simulink model "Group44VVI"  (R2022b)
settings: Solver=FixedStepAuto  StartTime=0.0  StopTime=10.0  FixedStep=1e-3  RelTol=1e-3  EnableMultiTasking=on
undefined symbols (not defined in the file): D1, D10, D11, D12, D2, D3, D4, D5, D7, D8, D9, PTA0, PTA1, PTA2, PTB23, PTB9, PTC17, PTC3, PTC4, PTD0, PTD2, PTD3
libraries: frdmk64flib x11
settings Model: ExtModeTrigDuration=5  Creator=Admin  LastModifiedBy=Admin
settings OptimizationCC: EnhancedBackFolding=on  PassReuseOutputArgsAs=Individual arguments  ZeroExternalMemoryAtStartup=off  ZeroInternalMemoryAtStartup=off  MaxStackSize=64  OptimizeBlockOrder=speed  DifferentSizesBufferReuse=on  OptimizationCustomize=off  EfficientTunableParamExpr=on
settings DebuggingCC: ParameterTunabilityLossMsg=error
settings HardwareCC: ProdBitPerPointer=32  ProdBitPerSizeT=32  ProdBitPerPtrDiffT=32  ProdLargestAtomicInteger=Long  ProdLargestAtomicFloat=Double  ProdWordSize=32  ProdHWDeviceType=ARM Compatible->ARM Cortex
settings SFSimCC: MATLABDynamicMemAlloc=off
settings RTWCC: Description=Embedded Coder  SystemTargetFile=ert.tlc  HardwareBoard=NXP FRDM-K64F  TLCOptions="-aInlineSetEventsForThisBaseRateFcn=TLC_FALSE -aSuppressMultiTaskScheduler=TLC_FALSE  -aRateBasedStepFcn=0"  TemplateMakefile=ert_default_tmf  Toolchain=GNU Tools for ARM Embedded Processors
settings CodeAppCC: ForceParamTrailComments=on  IgnoreCustomStorageClasses=off  OperatorAnnotations=on  SimulinkDataObjDesc=on  SFDataObjDesc=on  InsertBlockDesc=on
settings ERTTargetCC: ExtModeTransport=4  ExtModeMexFile=sendToCommService

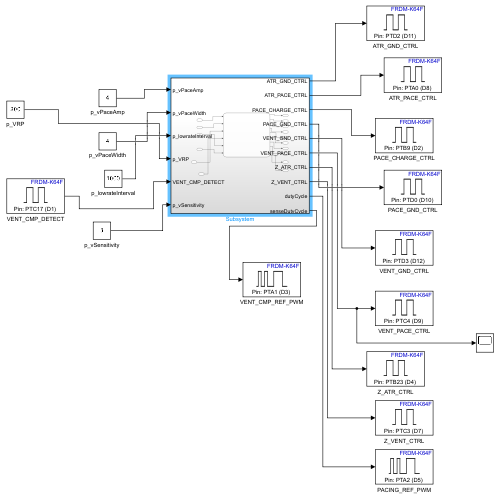
[thumbnail: Simulink's stored preview of the top-level diagram]
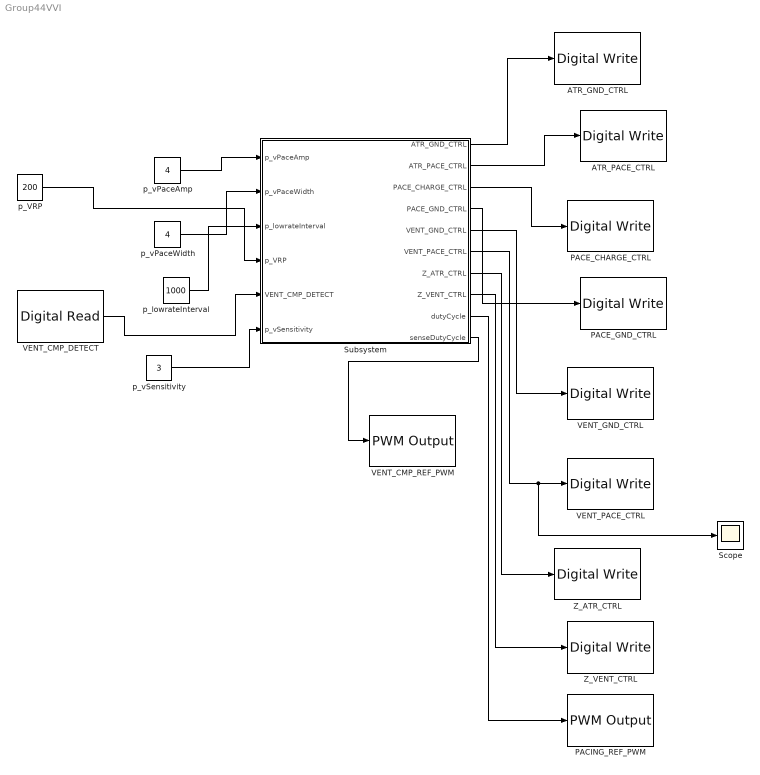
== system Group44VVI ==
  ATR_GND_CTRL : frdmk64flib/Digital Write  Whichpin=PTD2 (D11)
  ATR_PACE_CTRL : frdmk64flib/Digital Write  Whichpin=PTA0 (D8)
  PACE_CHARGE_CTRL : frdmk64flib/Digital Write  Whichpin=PTB9 (D2)
  PACE_GND_CTRL : frdmk64flib/Digital Write  Whichpin=PTD0 (D10)
  PACING_REF_PWM : frdmk64flib/PWM Output  Whichpin=PTA2 (D5)  InitialFrequency=2000  InitialDutyCycle=0
  Scope : Scope
  Subsystem : Subsystem
  VENT_CMP_DETECT : frdmk64flib/Digital Read  Whichpin=PTC17 (D1)  SampleTime=-1
  VENT_CMP_REF_PWM : frdmk64flib/PWM Output  Whichpin=PTA1 (D3)  InitialFrequency=2000  InitialDutyCycle=0
  VENT_GND_CTRL : frdmk64flib/Digital Write  Whichpin=PTD3 (D12)
  VENT_PACE_CTRL : frdmk64flib/Digital Write  Whichpin=PTC4 (D9)
  Z_ATR_CTRL : frdmk64flib/Digital Write  Whichpin=PTB23 (D4)
  Z_VENT_CTRL : frdmk64flib/Digital Write  Whichpin=PTC3 (D7)
  p_VRP : Constant  Value=200
  p_lowrateInterval : Constant  Value=1000  OutDataTypeStr=double
  p_vPaceAmp : Constant  Value=4  OutDataTypeStr=double
  p_vPaceWidth : Constant  Value=4  OutDataTypeStr=double
  p_vSensitivity : Constant  Value=3
  wires:
  p_vPaceWidth/1 -> Subsystem/2(p_vPaceWidth)
  Subsystem/5(VENT_GND_CTRL) -> VENT_GND_CTRL/1
  Subsystem/1(ATR_GND_CTRL) -> ATR_GND_CTRL/1
  Subsystem/6(VENT_PACE_CTRL) -> Scope/1, VENT_PACE_CTRL/1
  Subsystem/7(Z_ATR_CTRL) -> Z_ATR_CTRL/1
  p_VRP/1 -> Subsystem/4(p_VRP)
  p_vPaceAmp/1 -> Subsystem/1(p_vPaceAmp)
  Subsystem/2(ATR_PACE_CTRL) -> ATR_PACE_CTRL/1
  Subsystem/10(senseDutyCycle) -> VENT_CMP_REF_PWM/1
  Subsystem/4(PACE_GND_CTRL) -> PACE_GND_CTRL/1
  p_lowrateInterval/1 -> Subsystem/3(p_lowrateInterval)
  Subsystem/8(Z_VENT_CTRL) -> Z_VENT_CTRL/1
  Subsystem/3(PACE_CHARGE_CTRL) -> PACE_CHARGE_CTRL/1
  p_vSensitivity/1 -> Subsystem/6(p_vSensitivity)
  VENT_CMP_DETECT/1 -> Subsystem/5(VENT_CMP_DETECT)
  Subsystem/9(dutyCycle) -> PACING_REF_PWM/1

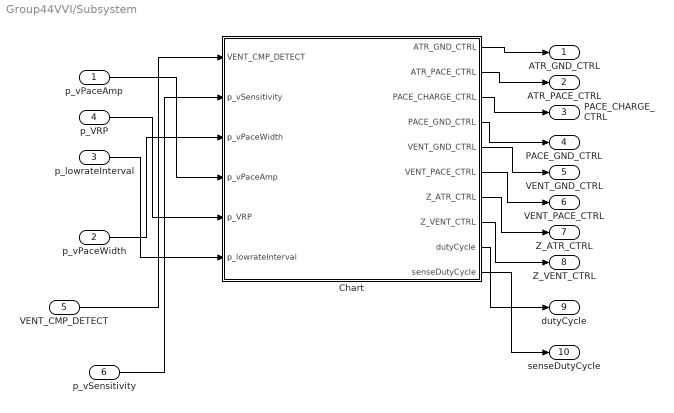
== system Group44VVI/Subsystem ==
  p_vPaceAmp : Inport
  p_vPaceWidth : Inport  Port=2
  p_lowrateInterval : Inport  Port=3
  p_VRP : Inport  Port=4
  VENT_CMP_DETECT : Inport  Port=5
  p_vSensitivity : Inport  Port=6
  Chart : Stateflow chart  TreatAsAtomicUnit=on
      settings: PortSchema="{\"entries\":[{\"content\":{\"sides\":[{\"content\":{\"connectorIds\":[\"In2\",\"In3\",\"In4\",\"In5\",\"In6\",\"In1\"]},\"type\":\"ConnectorPlacement.EquallySpacedRectSide\",\"uuid\":\"f4dc3048-51d6-4db6-b265-a066d0dfda2d\"},{\"content\":{\"connectorIds\":[\"Out1\",\"Out2\",\"Out3\",\"Out4\",\"Out5\",\"Out6\",\"Out7\",\"Out8\",\"Out9\",\"Out10\"],\"side\":\"RIGHT\"},\"type\":\"ConnectorPlacement.EquallySpacedRectSide\",\"uuid\":\"825f81e3-5cfe-4fd7-b9fc-d4806473552a\"},{\"content\":{\"connectorIds\":[],\"side\":\"TOP\"},\"type\":\"ConnectorPlacement.EquallySpacedRectSide\",\"uuid\":\"498485ba-e1f2-445a-9610-e3b27215c6f8\"}]},\"type\":\"ConnectorPlacement.EquallySpacedConnector\",\"uuid\":\"f957d02a-744b-46bb-8823-515c8e1b2a98\"}],\"packageUris\":[\"http://schema.mathworks.com/mf0/Connector/R2020b\"],\"version\":\"1.0\"}"
  ATR_GND_CTRL : Outport
  ATR_PACE_CTRL : Outport  Port=2
  PACE_CHARGE_CTRL : Outport  Port=3
  PACE_GND_CTRL : Outport  Port=4
  VENT_GND_CTRL : Outport  Port=5
  VENT_PACE_CTRL : Outport  Port=6
  Z_ATR_CTRL : Outport  Port=7
  Z_VENT_CTRL : Outport  Port=8
  dutyCycle : Outport  Port=9
  senseDutyCycle : Outport  Port=10
  wires:
  Chart/1(ATR_GND_CTRL) -> ATR_GND_CTRL/1
  Chart/2(ATR_PACE_CTRL) -> ATR_PACE_CTRL/1
  Chart/3(PACE_CHARGE_CTRL) -> PACE_CHARGE_CTRL/1
  Chart/4(PACE_GND_CTRL) -> PACE_GND_CTRL/1
  Chart/5(VENT_GND_CTRL) -> VENT_GND_CTRL/1
  Chart/6(VENT_PACE_CTRL) -> VENT_PACE_CTRL/1
  Chart/7(Z_ATR_CTRL) -> Z_ATR_CTRL/1
  Chart/8(Z_VENT_CTRL) -> Z_VENT_CTRL/1
  Chart/9(dutyCycle) -> dutyCycle/1
  Chart/10(senseDutyCycle) -> senseDutyCycle/1
  p_vPaceAmp/1 -> Chart/5(p_vPaceAmp)
  p_VRP/1 -> Chart/6(p_VRP)
  p_lowrateInterval/1 -> Chart/1(p_lowrateInterval)
  p_vPaceWidth/1 -> Chart/4(p_vPaceWidth)
  VENT_CMP_DETECT/1 -> Chart/2(VENT_CMP_DETECT)
  p_vSensitivity/1 -> Chart/3(p_vSensitivity)

== stateflow chart Group44VVI/Subsystem/Chart ==
  state ChargeC22_Atrial_DischargeC21
    entry:
    ATR_PACE_CTRL = false;
    VENT_PACE_CTRL = false;
    PACE_CHARGE_CTRL = true;
    PACE_GND_CTRL = true;
    Z_ATR_CTRL = false;
    Z_VENT_CTRL = false;
    ATR_GND_CTRL = false;
    VENT_GND_CTRL = true;
    dutyCycle=p_vPaceAmp/5.0*100
    senseDutyCycle = p_vSensitivity/5.0*100
  state PaceAtria
    entry:
    PACE_CHARGE_CTRL = false;
    PACE_GND_CTRL = true;
    ATR_PACE_CTRL = false;
    ATR_GND_CTRL = false;
    Z_ATR_CTRL = false;
    Z_VENT_CTRL = false;
    VENT_GND_CTRL = false;
    VENT_PACE_CTRL = true;
    %natPaceDetected=false;
  state AlertPeriod
  (default) -> ChargeC22_Atrial_DischargeC21
  PaceAtria -> ChargeC22_Atrial_DischargeC21 : after(p_vPaceWidth,msec)
  AlertPeriod -> PaceAtria [order 1] : after(p_lowrateInterval-p_vPaceWidth-p_VRP,msec)
  AlertPeriod -> ChargeC22_Atrial_DischargeC21 [order 2] : [VENT_CMP_DETECT == true ]
  ChargeC22_Atrial_DischargeC21 -> AlertPeriod : after(p_VRP,msec)
  data: p_lowrateInterval input; ATR_GND_CTRL output; ATR_PACE_CTRL output; PACE_CHARGE_CTRL output; PACE_GND_CTRL output; VENT_GND_CTRL output; VENT_PACE_CTRL output; Z_ATR_CTRL output; Z_VENT_CTRL output; dutyCycle output; senseDutyCycle output; VENT_CMP_DETECT input; p_vSensitivity input; p_vPaceWidth input; p_vPaceAmp input; p_VRP input
